simulink model "SAME5x_PIM_MCLV2_IOconfig"  (R2020b)
settings: Solver=FixedStepDiscrete  StartTime=0.0  StopTime=10.0  FixedStep=1e-4  MaxStep=1e-4  RelTol=1e-3  EnableMultiTasking=on
undefined symbols (not defined in the file): AIN0, AIN6, PA02, PA03, PA06, PA08, PA09, PA10, PA16, PA17, PA18, PB08, PC16, PC17, PC18, Pin, qdi0, qdi1, qdi2, SAME54P20A, Timer, TQFP128, VREFA, wo0, wo1, wo2, wo4, wo5, wo6
libraries: MCHP_Blockset x8, simulink x4, dsparch4 x1
(part 2 of 2)

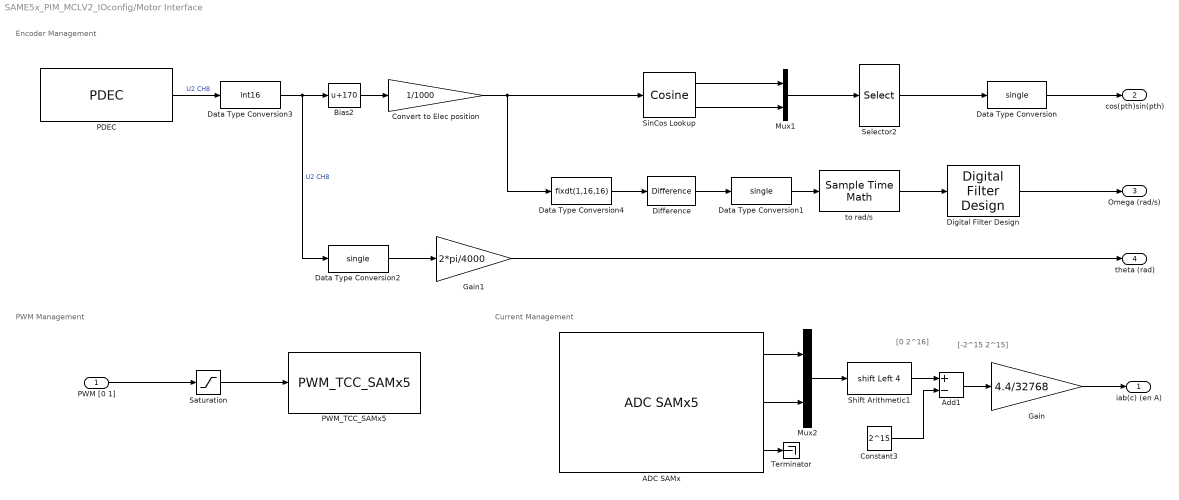
== system SAME5x_PIM_MCLV2_IOconfig/Motor Interface ==
  note: [-2^15 2^15]
  note: [0 2^16]
  note: Encoder Management
  note: PWM Management
  note: Current Management
  PWM [0 1] : Inport
  ADC SAMx : MCHP_Blockset/Analog IO/ADC SAMx5  ADCREF=ADC 0 and ADC 1 (slave)  VREF_seq0=PA03 / VREFA / Pin[10]  VREF_seq0_TXT=PA03 / VREFA / Pin[10]  info=0  SampleTime=1e-4  MCHP_PORT={ADC0_AIN1}{ADC0_AIN0}15:2:P2;{ADC0_AIN2}{ADC0_AIN6}15:2:P6;  MCHP_MASTERLINK=SAME5x_PIM_MCLV2_IOconfig/Microchip Master  ADC0_seq0=PA02 / AIN0 / Pin[9]  ADC0_seq0_TXT=PA02 / AIN0 / Pin[9]  ADC1_seq0=PB08 / AIN0 / Pin[19]  ADC1_seq0_TXT=PB08 / AIN0 / Pin[19]  Resolution_seq0=12 bits  SampleTime_seq0_s=1e-6  TrigSource_seq0=TCC0 PWM event Overflow  TrigTimeStep_seq0=on  ADC0_seq1=PA06 / AIN6 / Pin[23]  ADC0_seq1_TXT=PA06 / AIN6 / Pin[23]  ADC1_seq1=Not Used  ADC1_seq1_TXT=Not Used  Resolution_seq1=12 bits  SampleTime_seq1_s=1e-6  TrigSource_seq1=After previous sequence  TrigTimeStep_seq1=on
      settings: SourceProductName=MPLAB Device Blocks for Simulink
  Add1 : Sum  Inputs=+-  OutDataTypeStr=single
  Bias2 : Bias  Bias=170
  Constant3 : Constant  Value=2^15  OutDataTypeStr=fixdt(0,16,0)
  Convert to Elec position : Gain  Gain=1/1000  OutDataTypeStr=fixdt(0,16,16)
  Data Type Conversion : DataTypeConversion  OutDataTypeStr=single
  Data Type Conversion1 : DataTypeConversion  OutDataTypeStr=single
  Data Type Conversion2 : DataTypeConversion  OutDataTypeStr=single
  Data Type Conversion3 : DataTypeConversion  OutDataTypeStr=int16  ConvertRealWorld=Stored Integer (SI)
  Data Type Conversion4 : DataTypeConversion  OutDataTypeStr=fixdt(1,16,16)  ConvertRealWorld=Stored Integer (SI)
  Difference : simulink/Discrete/Difference  ICPrevInput=0  OutMin=[]  OutMax=[]  OutDataType=fixdt(1, 16)  OutScaling=2^-10  DoSatur=off
  Digital Filter Design : dsparch4/Digital Filter Design  mwdsp_browser_bugfix_var=off
  Gain : Gain  Gain=4.4/32768
  Gain1 : Gain  Gain=2*pi/4000
  Mux1 : Mux  Inputs=2
  Mux2 : Mux  Inputs=2
  PDEC : MCHP_Blockset/QEI/PDEC  Mode=Quadrature Encoder  index=Reset counter  QDI0=PC16 / Pin[70] / qdi0  QDI0_txt=Dynamic Options  QDI1=PC17 / Pin[71] / qdi1  QDI1_txt=Dynamic Options  QDI2=PC18 / Pin[72] / qdi2  QDI2_txt=Dynamic Options  maxCounterReset=-1  info=0  MCHP_MASTERLINK=SAME5x_PIM_MCLV2_IOconfig/Microchip Master  SampleTime=1e-4  MCHP_PORT={PDEC A}{PDEC_QDI0}5:0:P80;{PDEC B}{PDEC_QDI1}5:0:P81;{PDEC index}{PDEC_QDI2}5:0:P82;  MAXPOS_INPUT=off  RESET_INPUT=off  OutputCounter=on  OutputRevolution=off  CounterRevolution_length=Counter is 13 bits ; revolution is 3 bits  FILTER="250 (ns)  ->  freq 2 (MHz)"  FILTER_TXT="250 (ns)  ->  freq 2 (MHz)"  AutoCorrection=off  SWAP=off  QDI_invert_0=off  QDI_invert_1=off  QDI_invert_2=off
      settings: SourceProductName=MPLAB Device Blocks for Simulink
  PWM_TCC_SAMx5 : MCHP_Blockset/PWM IO/PWM_TCC_SAMx5  TCCREF=TCC 0  WAVE_choice=Center aligned PWM  MaxPeriod_s=5e-5  OTMX=Default  WO0=PA08 / Pin[33] / wo0  WO0_TXT=PA08 / Pin[33]  WO1=PA09 / Pin[34] / wo1  WO1_TXT=PA09 / Pin[34]  WO2=PA10 / Pin[35] / wo2  WO2_TXT=PA10 / Pin[35]  WO3=Not Used  WO3_TXT=Not Used  WO4=PA16 / Pin[66] / wo4  WO4_TXT=PA16 / Pin[66]  WO5=PA17 / Pin[67] / wo5  WO5_TXT=PA17 / Pin[67]  WO6=PA18 / Pin[68] / wo6  WO6_TXT=PA18 / Pin[68]  WO7=Not Used  WO7_TXT=Not Used  info=0  evalin_ws=PWM0max=MCHP_Fun.Hex2num('40A3860000000000');PWM0max=MCHP_Fun.Hex2num('40A3860000000000');PWM0max=MCHP_Fun.Hex2num('40A3860000000000');  SampleTime=1e-4  MCHP_PORT={PWM0_H0}{TCC0_WO0}5:1:P8;{PWM0_H1}{TCC0_WO1}5:1:P9;{PWM0_H2}{TCC0_WO2}5:1:P10;{PWM0_L0}{TCC0_WO4}5:1:P16;{PWM0_L1}{TCC0_WO5}5:1:P17;{PWM0_L2}{TCC0_WO6}5:1:P18;  MCHP_MASTERLINK=SAME5x_PIM_MCLV2_IOconfig/Microchip Master  INVEN_WO0=off  INVEN_WO1=off  INVEN_WO2=off  INVEN_WO3=off  INVEN_WO4=off  INVEN_WO5=off  INVEN_WO6=off  INVEN_WO7=off  SWAP_PWM0=off  SWAP_PWM1=off  SWAP_PWM2=off  SWAP_PWM3=off  POL_PWM0=off  POL_PWM1=off  POL_PWM2=off  POL_PWM3=off  POL_PWM4=off  POL_PWM5=off  InitPeriod_s=5e-5  InitDutyCycle_s=2.5e-5  InitDeadTimeH_s=0.5e-6  InitDeadTimeL_s=0.5e-6  BlockInput_VectorScalar=Vectors (grouped by function)  BlockInput_Period=Not a block input  BlockInput_DutyCycle=a Floating Point input within range [0 1]  BlockInput_DeadTime=Not a block input
      settings: SourceProductName=MPLAB Device Blocks for Simulink
  Saturation : Saturate  UpperLimit=0.98  LowerLimit=0.02  LinearizeAsGain=off  OutDataTypeStr=double
  Selector2 : Selector  InputPortWidth=2  IndexOptions=Index vector (dialog)  Indices=[2 1]  OutputSizes=1
  Shift Arithmetic1 : ArithShift  BitShiftNumber=4  BitShiftDirection=Left
  SinCos Lookup : simulink/Lookup Tables/Cosine  Formula=sin(2*pi*u) and cos(2*pi*u)  NumDataPoints=(2^12)+1  OutputWordLength=16  InternalRulePriority=Precision
      settings: SourceProductBaseCode=SL
  Terminator : Terminator
  to rad/s : SampleTimeMath  TsampMathOp=/  weightValue=4/(2*pi)
  iab(c) (en A) : Outport  VectorParamsAs1DForOutWhenUnconnected=off
  cos(pth)sin(pth) : Outport  Port=2  VectorParamsAs1DForOutWhenUnconnected=off
  Omega (rad/s) : Outport  Port=3  PortDimensions=1  VectorParamsAs1DForOutWhenUnconnected=off
  theta (rad) : Outport  Port=4  VectorParamsAs1DForOutWhenUnconnected=off
  wires:
  Saturation/1 -> PWM_TCC_SAMx5/1
  PWM [0 1]/1 -> Saturation/1
  ADC SAMx/1 -> Mux2/1
  ADC SAMx/2 -> Mux2/2
  Gain/1 -> iab(c) (en A)/1
  Shift Arithmetic1/1 -> Add1/1
  Mux2/1 -> Shift Arithmetic1/1
  Constant3/1 -> Add1/2
  Add1/1 -> Gain/1
  ADC SAMx/3 -> Terminator/1
  Data Type Conversion4/1 -> Difference/1
  Convert to Elec position/1 -> SinCos Lookup/1, Data Type Conversion4/1
  Data Type Conversion1/1 -> to rad/s/1
  to rad/s/1 -> Digital Filter Design/1
  Bias2/1 -> Convert to Elec position/1
  PDEC/1 -> Data Type Conversion3/1  "U2 CH8"
  Difference/1 -> Data Type Conversion1/1
  Digital Filter Design/1 -> Omega (rad/s)/1
  Data Type Conversion/1 -> cos(pth)sin(pth)/1
  Mux1/1 -> Selector2/1
  Selector2/1 -> Data Type Conversion/1
  SinCos Lookup/2 -> Mux1/2
  SinCos Lookup/1 -> Mux1/1
  Data Type Conversion3/1 -> Data Type Conversion2/1, Bias2/1  "U2 CH8"
  Data Type Conversion2/1 -> Gain1/1
  Gain1/1 -> theta (rad)/1
